simulink library "ProtoTrackDerivates"  (R2021a)
settings: Solver=VariableStepAuto  StartTime=0.0  StopTime=10.0  RelTol=1e-3
settings Model: Creator=z_zha  LastModifiedBy=z_zha

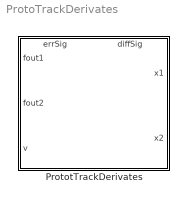
== system ProtoTrackDerivates ==
  PrototTrackDerivates : Subsystem  mask{R=300}
      mask prompts: R "Velocity factor'R'"
      settings: PortSchema="{\"entries\":[{\"content\":{\"sides\":[{\"content\":{\"connectorIds\":[\"In1\",\"In2\",\"In3\"]},\"type\":\"ConnectorPlacement.EquallySpacedRectSide\",\"uuid\":\"000cee14-9e68-449a-a4ac-67a7a3165385\"},{\"content\":{\"connectorIds\":[\"Out1\",\"Out2\"],\"side\":\"RIGHT\"},\"type\":\"ConnectorPlacement.EquallySpacedRectSide\",\"uuid\":\"72064135-bbc2-49e9-9ec1-0da547d5eb20\"},{\"content\":{\"connectorIds\":[\"Out3\",\"Out4\"],\"side\":\"TOP\"},\"type\":\"ConnectorPlacement.EquallySpacedRectSide\",\"uuid\":\"93e819c4-0116-4915-8c0a-583a4cdfd69c\"}]},\"type\":\"ConnectorPlacement.EquallySpacedConnector\",\"uuid\":\"23364127-30e4-4ddf-bda4-3f950a52342d\"}],\"packageUris\":[\"http://schema.mathworks.com/mf0/Connector/R2020b\"],\"version\":\"1.0\"}"

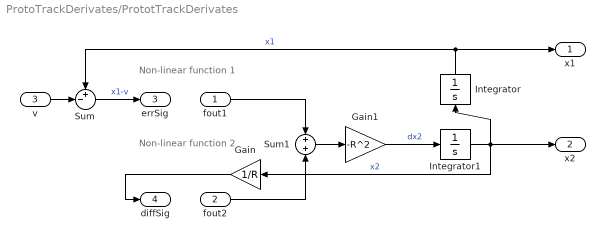
== system ProtoTrackDerivates/PrototTrackDerivates ==
  note: Non-linear function 1
  note: Non-linear function 2
  fout1 : Inport
  fout2 : Inport  Port=2
  v : Inport  Port=3
  Gain : Gain  Gain=1/R
  Gain1 : Gain  Gain=-R^2
  Integrator : Integrator
  Integrator1 : Integrator
  Sum : Sum  Inputs=+-|
  Sum1 : Sum  Inputs=+|+
  x1 : Outport  VectorParamsAs1DForOutWhenUnconnected=off
  x2 : Outport  Port=2  VectorParamsAs1DForOutWhenUnconnected=off
  errSig : Outport  Port=3
  diffSig : Outport  Port=4
  wires:
  fout1/1 -> Sum1/1
  fout2/1 -> Sum1/2
  Gain1/1 -> Integrator1/1  "dx2"
  v/1 -> Sum/2
  Integrator/1 -> Sum/1, x1/1  "x1"
  Sum1/1 -> Gain1/1
  Sum/1 -> errSig/1  "x1-v"
  Integrator1/1 -> Gain/1, Integrator/1, x2/1  "x2"
  Gain/1 -> diffSig/1
